simulink model "Per_MKM"  (R2019a)
settings: Solver=FixedStepDiscrete  StartTime=0.0  StopTime=50  FixedStep=1  RelTol=1e-3
undefined symbols (not defined in the file or in its folder): ADAS, ADAS_Setting, KeyPress, Setting
libraries: simulink x102
(part 1 of 2)
settings Model: DataDictionary=test2.sldd  Creator=admin  LastModifiedBy=inamdar
settings ConfigComp: CovMetricSettings=dtrzoibw  CovNameIncrementing=on  CovHtmlReporting=on  CovSaveCumulativeToWorkspaceVar=on  CovSaveSingleToWorkspaceVar=on  CovCumulativeReport=on

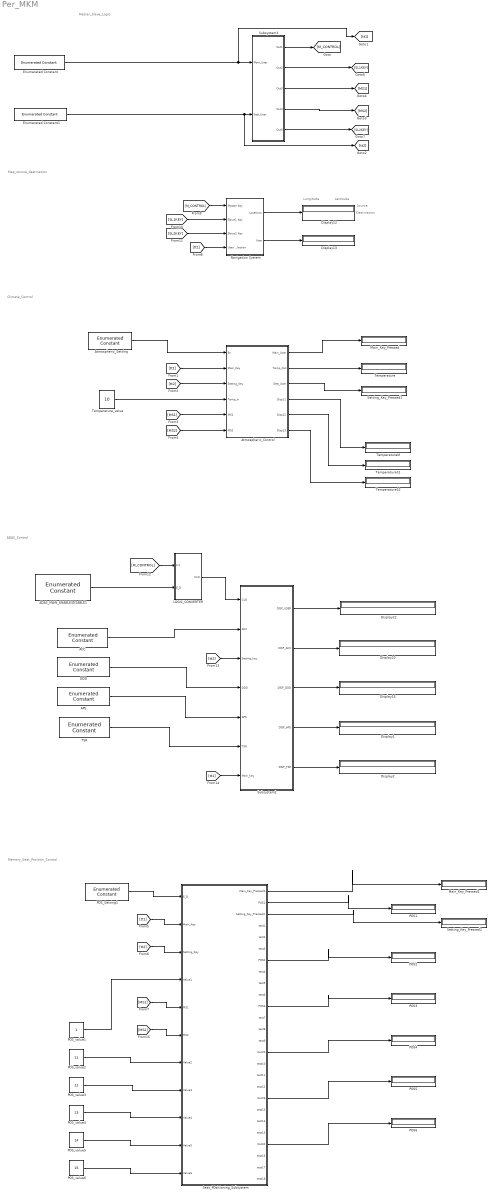
== system Per_MKM ==
  note: Memory_Seat_Position_Control
  note: Master_Slave_Logic
  note: Map_source_destination
  note: Climate_Control
  note: Longitude
  note: Lattitude
  note: Source
  note: Destination
  note: ADAS_Control
  ACC : simulink/Sources/Enumerated Constant  OutDataTypeStr=Enum: ADAS_Setting  Value=ADAS_Setting.Enable  SampleTime=inf
      settings: SourceProductName=Simulink
  ADAS_MAIN_ENABLE/DISABLE1 : simulink/Sources/Enumerated Constant  OutDataTypeStr=Enum: ADAS_Setting  Value=ADAS_Setting.Enable  SampleTime=inf
      settings: SourceProductName=Simulink
  APS : simulink/Sources/Enumerated Constant  OutDataTypeStr=Enum: ADAS_Setting  Value=ADAS_Setting.Enable  SampleTime=inf
      settings: SourceProductName=Simulink
  Atmospheric_Control : Subsystem
  Atmospheric_Setting : simulink/Sources/Enumerated Constant  OutDataTypeStr=Enum: Setting  Value=Setting.Disable  SampleTime=inf
      settings: SourceProductName=Simulink
  DDD : simulink/Sources/Enumerated Constant  OutDataTypeStr=Enum: ADAS_Setting  Value=ADAS_Setting.Enable  SampleTime=inf
      settings: SourceProductName=Simulink
  Display{1..2,12..14,20,22} (7 alike) : Display
  Enumerated Constant : simulink/Sources/Enumerated Constant  OutDataTypeStr=Enum: KeyPress  Value=KeyPress.Master  SampleTime=inf
      settings: SourceProductName=Simulink
  Enumerated Constant1 : simulink/Sources/Enumerated Constant  OutDataTypeStr=Enum: KeyPress  Value=KeyPress.Master  SampleTime=inf
      settings: SourceProductName=Simulink
  LOGIC_CONVERTER : Subsystem
  Main_Key_Pressed : Display
  Main_Key_Pressed1 : Display
  Navigation System : Subsystem
  POS{1..6} (6 alike) : Display
  POS_Setting1 : simulink/Sources/Enumerated Constant  OutDataTypeStr=Enum: Setting  Value=Setting.Disable  SampleTime=inf
      settings: SourceProductName=Simulink
  POS_value1 : Constant  OutDataTypeStr=uint8
  POS_value2 : Constant  Value=11  OutDataTypeStr=uint8
  POS_value3 : Constant  Value=12  OutDataTypeStr=uint8
  POS_value4 : Constant  Value=13  OutDataTypeStr=uint8
  POS_value5 : Constant  Value=14  OutDataTypeStr=uint8
  POS_value6 : Constant  Value=15  OutDataTypeStr=uint8
  Seat_POsitioning_Subsystem : Subsystem
  Setting_Key_Pressed1 : Display
  Setting_Key_Pressed2 : Display
  Subsystem2 : Subsystem
  Subsystem3 : Subsystem
  TSR : simulink/Sources/Enumerated Constant  OutDataTypeStr=Enum: ADAS_Setting  Value=ADAS_Setting.Enable  SampleTime=inf
      settings: SourceProductName=Simulink
  Temperature : Display
  TemperatureM : Display
  TemperatureS1 : Display
  TemperatureS2 : Display
  Temperature_value : Constant  Value=10  OutDataTypeStr=uint8
  wires:
  Enumerated Constant1/1 -> [tt2], Subsystem3/2(Sett_User)
  Navigation System/1(Locations) -> Display12/1
  Navigation System/2(User) -> Display13/1
  Enumerated Constant/1 -> [tt1], Subsystem3/1(Main_User)
  Atmospheric_Setting/1 -> Atmospheric_Control/1(En)
  [tt1] -> Atmospheric_Control/2(Main_Key)
  [tt2] -> Atmospheric_Control/3(Setting_Key)
  Temperature_value/1 -> Atmospheric_Control/4(Temp_In)
  Atmospheric_Control/1(Main_User) -> Main_Key_Pressed/1
  Atmospheric_Control/2(Temp_Out) -> Temperature/1
  Atmospheric_Control/3(Sett_User) -> Setting_Key_Pressed1/1
  [MS1] -> Atmospheric_Control/5("MS1 ")
  [MS2] -> Atmospheric_Control/6(MS2)
  [tt1] -> Navigation System/4(User Selection)
  [M_CONTROL] -> Navigation System/1("Master Key ")
  [SL1KEY] -> Navigation System/2(Slave1 Key)
  [SL2KEY] -> Navigation System/3(Slave2 Key)
  Subsystem2/5(DISP_TSR) -> Display2/1
  Subsystem2/4(DISP_APS) -> Display1/1
  Subsystem2/3(DISP_DDD) -> Display14/1
  Subsystem2/1(DISP_USER) -> Display22/1
  Subsystem2/2(DISP_ACC) -> Display20/1
  [tt1] -> Subsystem2/7(Main_key)
  TSR/1 -> Subsystem2/6(TSR)
  APS/1 -> Subsystem2/5(APS)
  DDD/1 -> Subsystem2/4(DDD)
  [tt2] -> Subsystem2/3(Setting_key)
  ACC/1 -> Subsystem2/2(ACC)
  [M_CONTROL] -> LOGIC_CONVERTER/1(In1)
  ADAS_MAIN_ENABLE/DISABLE1/1 -> LOGIC_CONVERTER/2(E_D)
  LOGIC_CONVERTER/1(CLO) -> Subsystem2/1(CLO)
  Subsystem3/1(Out1) -> [M_CONTROL]
  Subsystem3/2(Out2) -> [SL1KEY]
  Subsystem3/3(Out3) -> [MS1]
  Subsystem3/4(Out4) -> [MS2]
  Subsystem3/5(Out5) -> [SL2KEY]
  Atmospheric_Control/4(Disp11) -> TemperatureM/1
  Atmospheric_Control/5(Disp12) -> TemperatureS1/1
  Atmospheric_Control/6(Disp13) -> TemperatureS2/1
  POS_Setting1/1 -> Seat_POsitioning_Subsystem/1(E_D)
  [tt1] -> Seat_POsitioning_Subsystem/2(Main_Key)
  [tt2] -> Seat_POsitioning_Subsystem/3(Setting_Key)
  POS_value1/1 -> Seat_POsitioning_Subsystem/4(Value1)
  [MS1] -> Seat_POsitioning_Subsystem/5(MS1)
  [MS2] -> Seat_POsitioning_Subsystem/6(MS2)
  POS_value2/1 -> Seat_POsitioning_Subsystem/7(Value2)
  POS_value3/1 -> Seat_POsitioning_Subsystem/8(Value3)
  POS_value4/1 -> Seat_POsitioning_Subsystem/9(Value4)
  POS_value5/1 -> Seat_POsitioning_Subsystem/10(Value5)
  POS_value6/1 -> Seat_POsitioning_Subsystem/11(Value6)
  Seat_POsitioning_Subsystem/1(Main_Key_Pressed1) -> Main_Key_Pressed1/1
  Seat_POsitioning_Subsystem/2(POS1) -> POS1/1
  Seat_POsitioning_Subsystem/3(Setting_Key_Pressed2) -> Setting_Key_Pressed2/1
  Seat_POsitioning_Subsystem/7(POS2) -> POS2/1
  Seat_POsitioning_Subsystem/11(POS3) -> POS3/1
  Seat_POsitioning_Subsystem/15(Out20) -> POS4/1
  Seat_POsitioning_Subsystem/19(Out26) -> POS5/1
  Seat_POsitioning_Subsystem/23(Out32) -> POS6/1

== system Per_MKM/Atmospheric_Control ==
  En : Inport
  Main_Key : Inport  Port=2
  Setting_Key : Inport  Port=3
  Temp_In : Inport  Port=4
  "MS1 " : Inport  Port=5
  MS2 : Inport  Port=6
  Data Store Memory4 : DataStoreMemory  DataStoreName=TeM  ReadBeforeWriteMsg=warning  WriteAfterWriteMsg=warning  WriteAfterReadMsg=warning  ShowAdditionalParam=off  OutDataTypeStr=uint8
  Data Store Memory6 : DataStoreMemory  DataStoreName=TeS1  ReadBeforeWriteMsg=warning  WriteAfterWriteMsg=warning  WriteAfterReadMsg=warning  ShowAdditionalParam=off  OutDataTypeStr=uint8
  Data Store Memory7 : DataStoreMemory  DataStoreName=TeS2  ReadBeforeWriteMsg=warning  WriteAfterWriteMsg=warning  WriteAfterReadMsg=warning  ShowAdditionalParam=off  OutDataTypeStr=uint8
  Data Type Conversion1 : DataTypeConversion
  Data Type Conversion2 : DataTypeConversion
  Subsystem3 : Subsystem
  Subsystem4 : Subsystem
  Main_User : Outport
  Temp_Out : Outport  Port=2
  Sett_User : Outport  Port=3
  Disp11 : Outport  Port=4
  Disp12 : Outport  Port=5
  Disp13 : Outport  Port=6
  wires:
  Data Type Conversion2/1 -> Subsystem3/Enable
  Setting_Key/1 -> Subsystem3/1(In1)
  Subsystem4/1(Out1) -> Main_User/1
  Temp_In/1 -> Subsystem3/2(In2)
  Main_Key/1 -> Data Type Conversion1/1, Subsystem4/1(In1)
  Subsystem4/2(Out2) -> Temp_Out/1
  En/1 -> Data Type Conversion2/1
  MS2/1 -> Subsystem3/4(MS22)
  "MS1 "/1 -> Subsystem3/3(MS11)
  Subsystem3/1(Output) -> Sett_User/1
  Subsystem3/4(Disp3) -> Disp13/1
  Subsystem3/3(Disp2) -> Disp12/1
  Subsystem3/2(Disp1) -> Disp11/1
  Data Type Conversion1/1 -> Subsystem3/5(TT1)

== system Per_MKM/LOGIC_CONVERTER ==
  In1 : Inport
  E_D : Inport  Port=2
  AND1 : Logic  AllPortsSameDT=off  OutDataTypeStr=boolean
  Compare To Constant1 : simulink/Logic and Bit Operations/Compare To Constant  relop===  const=1  OutDataTypeStr=boolean
  Data Type Conversion2 : DataTypeConversion
  CLO : Outport
  wires:
  E_D/1 -> Data Type Conversion2/1
  Data Type Conversion2/1 -> Compare To Constant1/1
  Compare To Constant1/1 -> AND1/2
  In1/1 -> AND1/1
  AND1/1 -> CLO/1

== system Per_MKM/Navigation System ==
  "Master Key " : Inport
  Slave1 Key : Inport  Port=2
  Slave2 Key : Inport  Port=3
  User Selection : Inport  Port=4
  Subsystem2 : Subsystem
  Locations : Outport
  User : Outport  Port=2
  wires:
  "Master Key "/1 -> Subsystem2/1(In1)
  User Selection/1 -> User/1
  Slave1 Key/1 -> Subsystem2/2(In2)
  Slave2 Key/1 -> Subsystem2/3(In3)
  Subsystem2/1(Out1) -> Locations/1

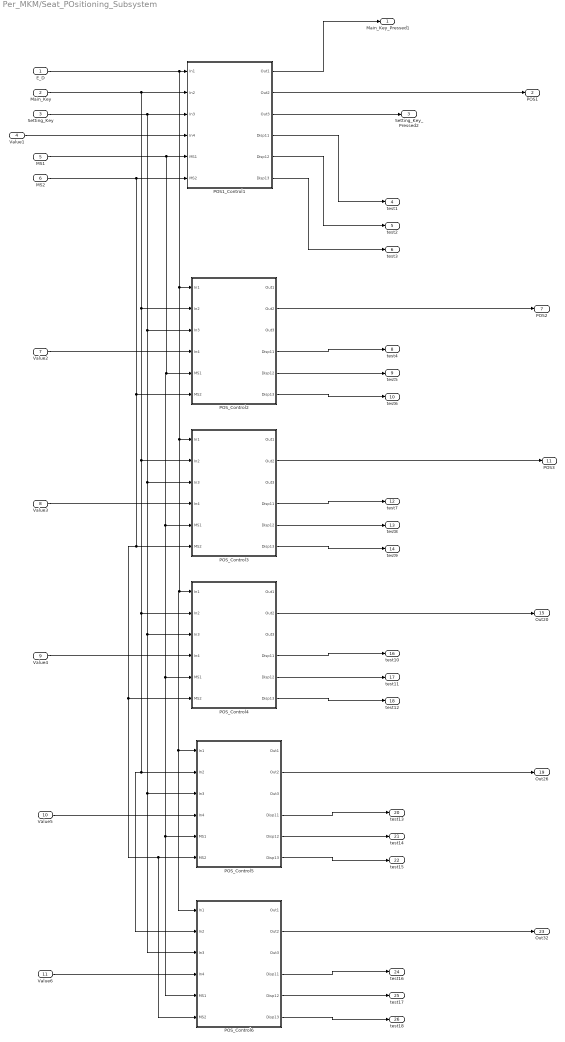
== system Per_MKM/Seat_POsitioning_Subsystem ==
  E_D : Inport
  Main_Key : Inport  Port=2
  Setting_Key : Inport  Port=3
  Value1 : Inport  Port=4
  MS1 : Inport  Port=5
  MS2 : Inport  Port=6
  Value2 : Inport  Port=7
  Value3 : Inport  Port=8
  Value4 : Inport  Port=9
  Value5 : Inport  Port=10
  Value6 : Inport  Port=11
  POS1_Control1 : Subsystem
  POS_Control2 : Subsystem
  POS_Control3 : Subsystem
  POS_Control4 : Subsystem
  POS_Control5 : Subsystem
  POS_Control6 : Subsystem
  Main_Key_Pressed1 : Outport
  POS1 : Outport  Port=2
  Setting_Key_Pressed2 : Outport  Port=3
  test1 : Outport  Port=4
  test2 : Outport  Port=5
  test3 : Outport  Port=6
  POS2 : Outport  Port=7
  test4 : Outport  Port=8
  test5 : Outport  Port=9
  test6 : Outport  Port=10
  POS3 : Outport  Port=11
  test7 : Outport  Port=12
  test8 : Outport  Port=13
  test9 : Outport  Port=14
  Out20 : Outport  Port=15
  test10 : Outport  Port=16
  test11 : Outport  Port=17
  test12 : Outport  Port=18
  Out26 : Outport  Port=19
  test13 : Outport  Port=20
  test14 : Outport  Port=21
  test15 : Outport  Port=22
  Out32 : Outport  Port=23
  test16 : Outport  Port=24
  test17 : Outport  Port=25
  test18 : Outport  Port=26
  wires:
  POS1_Control1/4(Disp11) -> test1/1
  MS1/1 -> POS_Control6/5("MS1 "), POS_Control5/5("MS1 "), POS_Control4/5("MS1 "), POS_Control3/5("MS1 "), POS_Control2/5("MS1 "), POS1_Control1/5("MS1 ")
  Setting_Key/1 -> POS_Control6/3(In3), POS_Control5/3(In3), POS_Control4/3(In3), POS_Control3/3(In3), POS_Control2/3(In3), POS1_Control1/3(In3)
  POS_Control3/4(Disp11) -> test7/1
  Main_Key/1 -> POS_Control6/2(In2), POS_Control5/2(In2), POS_Control4/2(In2), POS_Control3/2(In2), POS_Control2/2(In2), POS1_Control1/2(In2)
  E_D/1 -> POS_Control6/1(In1), POS_Control5/1(In1), POS_Control4/1(In1), POS_Control3/1(In1), POS_Control2/1(In1), POS1_Control1/1(In1)
  MS2/1 -> POS_Control6/6(MS2), POS_Control5/6(MS2), POS_Control4/6(MS2), POS_Control3/6(MS2), POS_Control2/6(MS2), POS1_Control1/6(MS2)
  Value1/1 -> POS1_Control1/4(In4)
  POS_Control6/4(Disp11) -> test16/1
  POS_Control3/6(Disp13) -> test9/1
  POS_Control3/2(Out2) -> POS3/1
  POS1_Control1/3(Out3) -> Setting_Key_Pressed2/1
  Value6/1 -> POS_Control6/4(In4)
  Value2/1 -> POS_Control2/4(In4)
  POS_Control2/5(Disp12) -> test5/1
  POS_Control2/6(Disp13) -> test6/1
  Value3/1 -> POS_Control3/4(In4)
  POS1_Control1/6(Disp13) -> test3/1
  POS1_Control1/1(Out1) -> Main_Key_Pressed1/1
  POS_Control5/5(Disp12) -> test14/1
  POS_Control5/6(Disp13) -> test15/1
  POS_Control2/2(Out2) -> POS2/1
  Value5/1 -> POS_Control5/4(In4)
  POS_Control2/4(Disp11) -> test4/1
  POS_Control3/5(Disp12) -> test8/1
  POS_Control4/4(Disp11) -> test10/1
  POS_Control4/5(Disp12) -> test11/1
  Value4/1 -> POS_Control4/4(In4)
  POS_Control6/5(Disp12) -> test17/1
  POS_Control4/6(Disp13) -> test12/1
  POS_Control5/2(Out2) -> Out26/1
  POS_Control4/2(Out2) -> Out20/1
  POS_Control6/6(Disp13) -> test18/1
  POS1_Control1/2(Out2) -> POS1/1
  POS_Control6/2(Out2) -> Out32/1
  POS1_Control1/5(Disp12) -> test2/1
  POS_Control5/4(Disp11) -> test13/1

== system Per_MKM/Subsystem2 ==
  CLO : Inport
  ACC : Inport  Port=2
  Setting_key : Inport  Port=3
  DDD : Inport  Port=4
  APS : Inport  Port=5
  TSR : Inport  Port=6
  Main_key : Inport  Port=7
  Data Store Memory : DataStoreMemory  DataStoreName=ADAS_M  ReadBeforeWriteMsg=warning  WriteAfterWriteMsg=warning  WriteAfterReadMsg=warning  ShowAdditionalParam=off
  Data Store Memory1 : DataStoreMemory  DataStoreName=ADAS_S1  ReadBeforeWriteMsg=warning  WriteAfterWriteMsg=warning  WriteAfterReadMsg=warning  ShowAdditionalParam=off
  Data Store Memory10 : DataStoreMemory  DataStoreName=ADAS_S13  ReadBeforeWriteMsg=warning  WriteAfterWriteMsg=warning  WriteAfterReadMsg=warning  ShowAdditionalParam=off
  Data Store Memory11 : DataStoreMemory  DataStoreName=ADAS_S23  ReadBeforeWriteMsg=warning  WriteAfterWriteMsg=warning  WriteAfterReadMsg=warning  ShowAdditionalParam=off
  Data Store Memory2 : DataStoreMemory  DataStoreName=ADAS_S2  ReadBeforeWriteMsg=warning  WriteAfterWriteMsg=warning  WriteAfterReadMsg=warning  ShowAdditionalParam=off
  Data Store Memory3 : DataStoreMemory  DataStoreName=ADAS_M1  ReadBeforeWriteMsg=warning  WriteAfterWriteMsg=warning  WriteAfterReadMsg=warning  ShowAdditionalParam=off
  Data Store Memory4 : DataStoreMemory  DataStoreName=ADAS_S11  ReadBeforeWriteMsg=warning  WriteAfterWriteMsg=warning  WriteAfterReadMsg=warning  ShowAdditionalParam=off
  Data Store Memory5 : DataStoreMemory  DataStoreName=ADAS_S21  ReadBeforeWriteMsg=warning  WriteAfterWriteMsg=warning  WriteAfterReadMsg=warning  ShowAdditionalParam=off
  Data Store Memory6 : DataStoreMemory  DataStoreName=ADAS_M2  ReadBeforeWriteMsg=warning  WriteAfterWriteMsg=warning  WriteAfterReadMsg=warning  ShowAdditionalParam=off
  Data Store Memory7 : DataStoreMemory  DataStoreName=ADAS_S12  ReadBeforeWriteMsg=warning  WriteAfterWriteMsg=warning  WriteAfterReadMsg=warning  ShowAdditionalParam=off
  Data Store Memory8 : DataStoreMemory  DataStoreName=ADAS_S22  ReadBeforeWriteMsg=warning  WriteAfterWriteMsg=warning  WriteAfterReadMsg=warning  ShowAdditionalParam=off
  Data Store Memory9 : DataStoreMemory  DataStoreName=ADAS_M3  ReadBeforeWriteMsg=warning  WriteAfterWriteMsg=warning  WriteAfterReadMsg=warning  ShowAdditionalParam=off
  Subsystem : Subsystem
  Subsystem1 : Subsystem
  Subsystem8 : Subsystem
  DISP_USER : Outport
  DISP_ACC : Outport  Port=2
  DISP_DDD : Outport  Port=3
  DISP_APS : Outport  Port=4
  DISP_TSR : Outport  Port=5
  wires:
  CLO/1 -> Subsystem8/Enable, [LOGIC_DISPLAY]
  TSR/1 -> Subsystem8/5(In5)
  APS/1 -> Subsystem8/4(In4)
  DDD/1 -> Subsystem8/3(In3)
  Setting_key/1 -> Subsystem8/2(In2)
  ACC/1 -> Subsystem8/1(In1)
  Main_key/1 -> Subsystem/1(In1), Subsystem1/7(In7)
  Subsystem8/1(Out1) -> Subsystem1/1(In1)
  [LOGIC_DISPLAY] -> Subsystem1/2(In2)
  Subsystem8/2(Out2) -> Subsystem1/3(In3)
  Subsystem8/3(Out3) -> Subsystem1/4(In4)
  Subsystem8/4(Out4) -> Subsystem1/5(In5)
  Subsystem8/5(Out5) -> Subsystem1/6(In6)
  Subsystem/1(Out1) -> Subsystem1/8(In8)
  Subsystem/2(Out2) -> Subsystem1/9(In9)
  Subsystem/3(Out3) -> Subsystem1/10(In10)
  Subsystem/4(Out4) -> Subsystem1/11(In11)
  Subsystem1/1(Out1) -> DISP_USER/1
  Subsystem1/2(Out2) -> DISP_ACC/1
  Subsystem1/3(Out3) -> DISP_DDD/1
  Subsystem1/4(Out4) -> DISP_APS/1
  Subsystem1/5(Out5) -> DISP_TSR/1

== system Per_MKM/Subsystem3 ==
  Main_User : Inport
  Sett_User : Inport  Port=2
  Logics : Subsystem
  Subsystem : Subsystem
  Subsystem1 : Subsystem
  Out1 : Outport
  Out2 : Outport  Port=2
  Out3 : Outport  Port=3
  Out4 : Outport  Port=4
  Out5 : Outport  Port=5
  wires:
  Subsystem1/2(Out3) -> Logics/3(In5)
  Logics/1(Out2) -> Out3/1
  Subsystem1/1(Out2) -> Logics/2(In4)
  Subsystem/2(Out3) -> Out2/1
  Subsystem/3(Out4) -> Out5/1
  Subsystem1/3(Out4) -> Logics/4(In6)
  Subsystem/1(Out2) -> Out1/1, Logics/1(In1)
  Logics/2(Out3) -> Out4/1
  Sett_User/1 -> Subsystem1/1(In1)
  Main_User/1 -> Subsystem/1(In1)

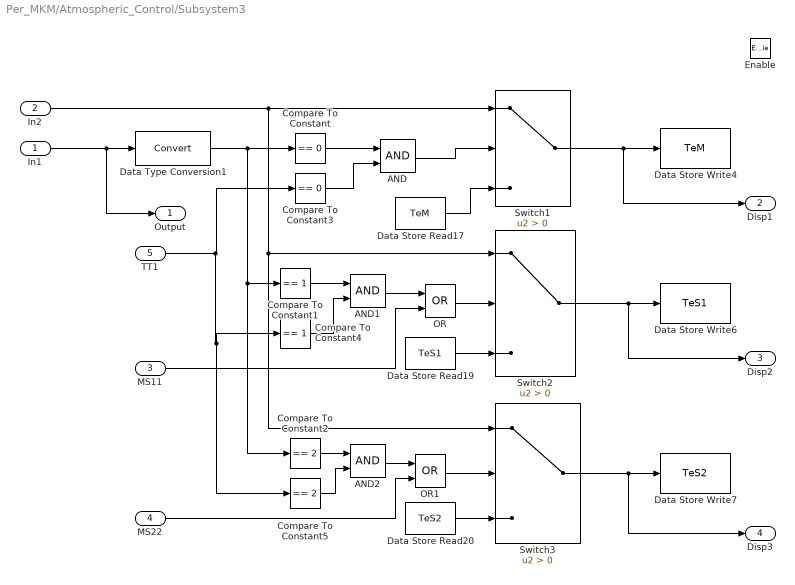
== system Per_MKM/Atmospheric_Control/Subsystem3 ==
  In1 : Inport
  In2 : Inport  Port=2
  MS11 : Inport  Port=3
  MS22 : Inport  Port=4
  TT1 : Inport  Port=5
  Enable : EnablePort
  AND : Logic  AllPortsSameDT=off  OutDataTypeStr=boolean
  AND1 : Logic  AllPortsSameDT=off  OutDataTypeStr=boolean
  AND2 : Logic  AllPortsSameDT=off  OutDataTypeStr=boolean
  Compare To Constant : simulink/Logic and Bit Operations/Compare To Constant  relop===  const=0  OutDataTypeStr=boolean
  Compare To Constant1 : simulink/Logic and Bit Operations/Compare To Constant  relop===  const=1  OutDataTypeStr=boolean
  Compare To Constant2 : simulink/Logic and Bit Operations/Compare To Constant  relop===  const=2  OutDataTypeStr=boolean
  Compare To Constant3 : simulink/Logic and Bit Operations/Compare To Constant  relop===  const=0  OutDataTypeStr=boolean
  Compare To Constant4 : simulink/Logic and Bit Operations/Compare To Constant  relop===  const=1  OutDataTypeStr=boolean
  Compare To Constant5 : simulink/Logic and Bit Operations/Compare To Constant  relop===  const=2  OutDataTypeStr=boolean
  Data Store Read17 : DataStoreRead  DataStoreName=TeM
  Data Store Read19 : DataStoreRead  DataStoreName=TeS1
  Data Store Read20 : DataStoreRead  DataStoreName=TeS2
  Data Store Write4 : DataStoreWrite  DataStoreName=TeM
  Data Store Write6 : DataStoreWrite  DataStoreName=TeS1
  Data Store Write7 : DataStoreWrite  DataStoreName=TeS2
  Data Type Conversion1 : DataTypeConversion
  OR : Logic  Operator=OR  AllPortsSameDT=off  OutDataTypeStr=boolean
  OR1 : Logic  Operator=OR  AllPortsSameDT=off  OutDataTypeStr=boolean
  Switch1 : Switch  Criteria=u2 > Threshold
  Switch2 : Switch  Criteria=u2 > Threshold
  Switch3 : Switch  Criteria=u2 > Threshold
  Output : Outport
  Disp1 : Outport  Port=2
  Disp2 : Outport  Port=3
  Disp3 : Outport  Port=4
  wires:
  Data Type Conversion1/1 -> Compare To Constant/1, Compare To Constant2/1, Compare To Constant1/1
  Switch2/1 -> Disp2/1, Data Store Write6/1
  Data Store Read20/1 -> Switch3/3
  Switch3/1 -> Disp3/1, Data Store Write7/1
  Switch1/1 -> Disp1/1, Data Store Write4/1
  Data Store Read19/1 -> Switch2/3
  Data Store Read17/1 -> Switch1/3
  In1/1 -> Output/1, Data Type Conversion1/1
  In2/1 -> Switch1/1, Switch2/1, Switch3/1
  OR/1 -> Switch2/2
  OR1/1 -> Switch3/2
  MS11/1 -> OR/2
  MS22/1 -> OR1/2
  AND/1 -> Switch1/2
  Compare To Constant/1 -> AND/1
  Compare To Constant3/1 -> AND/2
  TT1/1 -> Compare To Constant5/1, Compare To Constant4/1, Compare To Constant3/1
  Compare To Constant1/1 -> AND1/1
  Compare To Constant4/1 -> AND1/2
  AND1/1 -> OR/1
  AND2/1 -> OR1/1
  Compare To Constant2/1 -> AND2/1
  Compare To Constant5/1 -> AND2/2

== system Per_MKM/Atmospheric_Control/Subsystem4 ==
  In1 : Inport
  Data Store Read14 : DataStoreRead  DataStoreName=TeM
  Data Store Read15 : DataStoreRead  DataStoreName=TeS1
  Data Store Read16 : DataStoreRead  DataStoreName=TeS2
  Data Type Conversion : DataTypeConversion
  Multiport Switch3 : MultiPortSwitch  DataPortOrder=Zero-based contiguous  DataPortForDefault=Additional data port  zeroidx=on
  Out1 : Outport
  Out2 : Outport  Port=2
  wires:
  In1/1 -> Out1/1, Data Type Conversion/1
  Data Store Read14/1 -> Multiport Switch3/5, Multiport Switch3/2
  Multiport Switch3/1 -> Out2/1
  Data Type Conversion/1 -> Multiport Switch3/1
  Data Store Read15/1 -> Multiport Switch3/3
  Data Store Read16/1 -> Multiport Switch3/4

== system Per_MKM/Navigation System/Subsystem2 ==
  In1 : Inport
  In2 : Inport  Port=2
  In3 : Inport  Port=3
  Constant10 : Constant  Value=0
  Constant6 : Constant  Value=[18.6 73.75]
  Constant7 : Constant  Value=[18.44 73.86]
  Constant8 : Constant  Value=[ 18.43 73.77]
  Constant9 : Constant  Value=[18.53 73.87]
  Mux : Mux  Inputs=2
  Switch1 : Switch  Criteria=u2 > Threshold
  Switch2 : Switch  Criteria=u2 > Threshold
  Switch3 : Switch  Criteria=u2 > Threshold
  Out1 : Outport
  wires:
  Switch2/1 -> Switch1/3
  Constant7/1 -> Switch2/1
  Switch3/1 -> Switch2/3
  Constant9/1 -> Switch1/1
  Constant8/1 -> Switch3/1
  Constant6/1 -> Mux/1
  Switch1/1 -> Mux/2
  Constant10/1 -> Switch3/3
  In3/1 -> Switch3/2
  In2/1 -> Switch2/2
  In1/1 -> Switch1/2
  Mux/1 -> Out1/1

== system Per_MKM/Seat_POsitioning_Subsystem/POS1_Control1 ==
  In1 : Inport
  In2 : Inport  Port=2
  In3 : Inport  Port=3
  In4 : Inport  Port=4
  "MS1 " : Inport  Port=5
  MS2 : Inport  Port=6
  Data Store Memory4 : DataStoreMemory  DataStoreName=POS_M  ReadBeforeWriteMsg=warning  WriteAfterWriteMsg=warning  WriteAfterReadMsg=warning  ShowAdditionalParam=off  OutDataTypeStr=uint8
  Data Store Memory6 : DataStoreMemory  DataStoreName=POS_S1  ReadBeforeWriteMsg=warning  WriteAfterWriteMsg=warning  WriteAfterReadMsg=warning  ShowAdditionalParam=off  OutDataTypeStr=uint8
  Data Store Memory7 : DataStoreMemory  DataStoreName=POS_S2  ReadBeforeWriteMsg=warning  WriteAfterWriteMsg=warning  WriteAfterReadMsg=warning  ShowAdditionalParam=off  OutDataTypeStr=uint8
  Data Type Conversion1 : DataTypeConversion
  Data Type Conversion2 : DataTypeConversion
  Subsystem3 : Subsystem
  Subsystem4 : Subsystem
  Out1 : Outport
  Out2 : Outport  Port=2
  Out3 : Outport  Port=3
  Disp11 : Outport  Port=4
  Disp12 : Outport  Port=5
  Disp13 : Outport  Port=6
  wires:
  Data Type Conversion1/1 -> Subsystem3/5(TT1)
  Subsystem3/2(Disp1) -> Disp11/1
  Subsystem3/3(Disp2) -> Disp12/1
  Subsystem3/4(Disp3) -> Disp13/1
  Subsystem3/1(Output) -> Out3/1
  "MS1 "/1 -> Subsystem3/3(MS11)
  MS2/1 -> Subsystem3/4(MS22)
  In1/1 -> Data Type Conversion2/1
  Subsystem4/2(Out2) -> Out2/1
  In2/1 -> Subsystem4/1(In1), Data Type Conversion1/1
  In4/1 -> Subsystem3/2(In2)
  Subsystem4/1(Out1) -> Out1/1
  In3/1 -> Subsystem3/1(In1)
  Data Type Conversion2/1 -> Subsystem3/Enable

== system Per_MKM/Seat_POsitioning_Subsystem/POS_Control2 ==
  In1 : Inport
  In2 : Inport  Port=2
  In3 : Inport  Port=3
  In4 : Inport  Port=4
  "MS1 " : Inport  Port=5
  MS2 : Inport  Port=6
  Data Store Memory4 : DataStoreMemory  DataStoreName=POS_M1  ReadBeforeWriteMsg=warning  WriteAfterWriteMsg=warning  WriteAfterReadMsg=warning  ShowAdditionalParam=off  OutDataTypeStr=uint8
  Data Store Memory6 : DataStoreMemory  DataStoreName=POS_S11  ReadBeforeWriteMsg=warning  WriteAfterWriteMsg=warning  WriteAfterReadMsg=warning  ShowAdditionalParam=off  OutDataTypeStr=uint8
  Data Store Memory7 : DataStoreMemory  DataStoreName=POS_S21  ReadBeforeWriteMsg=warning  WriteAfterWriteMsg=warning  WriteAfterReadMsg=warning  ShowAdditionalParam=off  OutDataTypeStr=uint8
  Data Type Conversion1 : DataTypeConversion
  Data Type Conversion2 : DataTypeConversion
  Subsystem3 : Subsystem
  Subsystem4 : Subsystem
  Out1 : Outport
  Out2 : Outport  Port=2
  Out3 : Outport  Port=3
  Disp11 : Outport  Port=4
  Disp12 : Outport  Port=5
  Disp13 : Outport  Port=6
  wires:
  Data Type Conversion2/1 -> Subsystem3/Enable
  In3/1 -> Subsystem3/1(In1)
  Subsystem4/1(Out1) -> Out1/1
  In4/1 -> Subsystem3/2(In2)
  In2/1 -> Data Type Conversion1/1, Subsystem4/1(In1)
  Subsystem4/2(Out2) -> Out2/1
  In1/1 -> Data Type Conversion2/1
  MS2/1 -> Subsystem3/4(MS22)
  "MS1 "/1 -> Subsystem3/3(MS11)
  Subsystem3/1(Output) -> Out3/1
  Subsystem3/4(Disp3) -> Disp13/1
  Subsystem3/3(Disp2) -> Disp12/1
  Subsystem3/2(Disp1) -> Disp11/1
  Data Type Conversion1/1 -> Subsystem3/5(TT1)

== system Per_MKM/Seat_POsitioning_Subsystem/POS_Control3 ==
  In1 : Inport
  In2 : Inport  Port=2
  In3 : Inport  Port=3
  In4 : Inport  Port=4
  "MS1 " : Inport  Port=5
  MS2 : Inport  Port=6
  Data Store Memory4 : DataStoreMemory  DataStoreName=POS_M11  ReadBeforeWriteMsg=warning  WriteAfterWriteMsg=warning  WriteAfterReadMsg=warning  ShowAdditionalParam=off  OutDataTypeStr=uint8
  Data Store Memory6 : DataStoreMemory  DataStoreName=POS_S111  ReadBeforeWriteMsg=warning  WriteAfterWriteMsg=warning  WriteAfterReadMsg=warning  ShowAdditionalParam=off  OutDataTypeStr=uint8
  Data Store Memory7 : DataStoreMemory  DataStoreName=POS_S211  ReadBeforeWriteMsg=warning  WriteAfterWriteMsg=warning  WriteAfterReadMsg=warning  ShowAdditionalParam=off  OutDataTypeStr=uint8
  Data Type Conversion1 : DataTypeConversion
  Data Type Conversion2 : DataTypeConversion
  Subsystem3 : Subsystem
  Subsystem4 : Subsystem
  Out1 : Outport
  Out2 : Outport  Port=2
  Out3 : Outport  Port=3
  Disp11 : Outport  Port=4
  Disp12 : Outport  Port=5
  Disp13 : Outport  Port=6
  wires:
  Data Type Conversion1/1 -> Subsystem3/5(TT1)
  Subsystem3/2(Disp1) -> Disp11/1
  Subsystem3/3(Disp2) -> Disp12/1
  Subsystem3/4(Disp3) -> Disp13/1
  Subsystem3/1(Output) -> Out3/1
  "MS1 "/1 -> Subsystem3/3(MS11)
  MS2/1 -> Subsystem3/4(MS22)
  In1/1 -> Data Type Conversion2/1
  Subsystem4/2(Out2) -> Out2/1
  In2/1 -> Subsystem4/1(In1), Data Type Conversion1/1
  In4/1 -> Subsystem3/2(In2)
  Subsystem4/1(Out1) -> Out1/1
  In3/1 -> Subsystem3/1(In1)
  Data Type Conversion2/1 -> Subsystem3/Enable

== system Per_MKM/Seat_POsitioning_Subsystem/POS_Control4 ==
  In1 : Inport
  In2 : Inport  Port=2
  In3 : Inport  Port=3
  In4 : Inport  Port=4
  "MS1 " : Inport  Port=5
  MS2 : Inport  Port=6
  Data Store Memory4 : DataStoreMemory  DataStoreName=POS_M4  ReadBeforeWriteMsg=warning  WriteAfterWriteMsg=warning  WriteAfterReadMsg=warning  ShowAdditionalParam=off  OutDataTypeStr=uint8
  Data Store Memory6 : DataStoreMemory  DataStoreName=POS_S14  ReadBeforeWriteMsg=warning  WriteAfterWriteMsg=warning  WriteAfterReadMsg=warning  ShowAdditionalParam=off  OutDataTypeStr=uint8
  Data Store Memory7 : DataStoreMemory  DataStoreName=POS_S24  ReadBeforeWriteMsg=warning  WriteAfterWriteMsg=warning  WriteAfterReadMsg=warning  ShowAdditionalParam=off  OutDataTypeStr=uint8
  Data Type Conversion1 : DataTypeConversion
  Data Type Conversion2 : DataTypeConversion
  Subsystem3 : Subsystem
  Subsystem4 : Subsystem
  Out1 : Outport
  Out2 : Outport  Port=2
  Out3 : Outport  Port=3
  Disp11 : Outport  Port=4
  Disp12 : Outport  Port=5
  Disp13 : Outport  Port=6
  wires:
  Data Type Conversion2/1 -> Subsystem3/Enable
  In3/1 -> Subsystem3/1(In1)
  Subsystem4/1(Out1) -> Out1/1
  In4/1 -> Subsystem3/2(In2)
  In2/1 -> Data Type Conversion1/1, Subsystem4/1(In1)
  Subsystem4/2(Out2) -> Out2/1
  In1/1 -> Data Type Conversion2/1
  MS2/1 -> Subsystem3/4(MS22)
  "MS1 "/1 -> Subsystem3/3(MS11)
  Subsystem3/1(Output) -> Out3/1
  Subsystem3/4(Disp3) -> Disp13/1
  Subsystem3/3(Disp2) -> Disp12/1
  Subsystem3/2(Disp1) -> Disp11/1
  Data Type Conversion1/1 -> Subsystem3/5(TT1)

== system Per_MKM/Seat_POsitioning_Subsystem/POS_Control5 ==
  In1 : Inport
  In2 : Inport  Port=2
  In3 : Inport  Port=3
  In4 : Inport  Port=4
  "MS1 " : Inport  Port=5
  MS2 : Inport  Port=6
  Data Store Memory4 : DataStoreMemory  DataStoreName=POS_M5  ReadBeforeWriteMsg=warning  WriteAfterWriteMsg=warning  WriteAfterReadMsg=warning  ShowAdditionalParam=off  OutDataTypeStr=uint8
  Data Store Memory6 : DataStoreMemory  DataStoreName=POS_S15  ReadBeforeWriteMsg=warning  WriteAfterWriteMsg=warning  WriteAfterReadMsg=warning  ShowAdditionalParam=off  OutDataTypeStr=uint8
  Data Store Memory7 : DataStoreMemory  DataStoreName=POS_S25  ReadBeforeWriteMsg=warning  WriteAfterWriteMsg=warning  WriteAfterReadMsg=warning  ShowAdditionalParam=off  OutDataTypeStr=uint8
  Data Type Conversion1 : DataTypeConversion
  Data Type Conversion2 : DataTypeConversion
  Subsystem3 : Subsystem
  Subsystem4 : Subsystem
  Out1 : Outport
  Out2 : Outport  Port=2
  Out3 : Outport  Port=3
  Disp11 : Outport  Port=4
  Disp12 : Outport  Port=5
  Disp13 : Outport  Port=6
  wires:
  Data Type Conversion1/1 -> Subsystem3/5(TT1)
  Subsystem3/2(Disp1) -> Disp11/1
  Subsystem3/3(Disp2) -> Disp12/1
  Subsystem3/4(Disp3) -> Disp13/1
  Subsystem3/1(Output) -> Out3/1
  "MS1 "/1 -> Subsystem3/3(MS11)
  MS2/1 -> Subsystem3/4(MS22)
  In1/1 -> Data Type Conversion2/1
  Subsystem4/2(Out2) -> Out2/1
  In2/1 -> Subsystem4/1(In1), Data Type Conversion1/1
  In4/1 -> Subsystem3/2(In2)
  Subsystem4/1(Out1) -> Out1/1
  In3/1 -> Subsystem3/1(In1)
  Data Type Conversion2/1 -> Subsystem3/Enable

== system Per_MKM/Seat_POsitioning_Subsystem/POS_Control6 ==
  In1 : Inport
  In2 : Inport  Port=2
  In3 : Inport  Port=3
  In4 : Inport  Port=4
  "MS1 " : Inport  Port=5
  MS2 : Inport  Port=6
  Data Store Memory4 : DataStoreMemory  DataStoreName=POS_M6  ReadBeforeWriteMsg=warning  WriteAfterWriteMsg=warning  WriteAfterReadMsg=warning  ShowAdditionalParam=off  OutDataTypeStr=uint8
  Data Store Memory6 : DataStoreMemory  DataStoreName=POS_S16  ReadBeforeWriteMsg=warning  WriteAfterWriteMsg=warning  WriteAfterReadMsg=warning  ShowAdditionalParam=off  OutDataTypeStr=uint8
  Data Store Memory7 : DataStoreMemory  DataStoreName=POS_S26  ReadBeforeWriteMsg=warning  WriteAfterWriteMsg=warning  WriteAfterReadMsg=warning  ShowAdditionalParam=off  OutDataTypeStr=uint8
  Data Type Conversion1 : DataTypeConversion
  Data Type Conversion2 : DataTypeConversion
  Subsystem3 : Subsystem
  Subsystem4 : Subsystem
  Out1 : Outport
  Out2 : Outport  Port=2
  Out3 : Outport  Port=3
  Disp11 : Outport  Port=4
  Disp12 : Outport  Port=5
  Disp13 : Outport  Port=6
  wires:
  Data Type Conversion2/1 -> Subsystem3/Enable
  In3/1 -> Subsystem3/1(In1)
  Subsystem4/1(Out1) -> Out1/1
  In4/1 -> Subsystem3/2(In2)
  In2/1 -> Data Type Conversion1/1, Subsystem4/1(In1)
  Subsystem4/2(Out2) -> Out2/1
  In1/1 -> Data Type Conversion2/1
  MS2/1 -> Subsystem3/4(MS22)
  "MS1 "/1 -> Subsystem3/3(MS11)
  Subsystem3/1(Output) -> Out3/1
  Subsystem3/4(Disp3) -> Disp13/1
  Subsystem3/3(Disp2) -> Disp12/1
  Subsystem3/2(Disp1) -> Disp11/1
  Data Type Conversion1/1 -> Subsystem3/5(TT1)

== system Per_MKM/Subsystem2/Subsystem ==
  In1 : Inport
  Subsystem_ACC : Subsystem
  Subsystem_APSD : Subsystem
  Subsystem_DDDE : Subsystem
  Subsystem_TSRC : Subsystem
  Out1 : Outport
  Out2 : Outport  Port=2
  Out3 : Outport  Port=3
  Out4 : Outport  Port=4
  wires:
  Subsystem_ACC/1(Out1) -> Out1/1
  In1/1 -> Subsystem_TSRC/1(In1), Subsystem_APSD/1(In1), Subsystem_DDDE/1(In1), Subsystem_ACC/1(In1)
  Subsystem_DDDE/1(Out1) -> Out2/1
  Subsystem_APSD/1(Out1) -> Out3/1
  Subsystem_TSRC/1(Out1) -> Out4/1

== system Per_MKM/Subsystem2/Subsystem1 ==
  In1 : Inport
  In2 : Inport  Port=2
  In3 : Inport  Port=3
  In4 : Inport  Port=4
  In5 : Inport  Port=5
  In6 : Inport  Port=6
  In7 : Inport  Port=7
  In8 : Inport  Port=8
  In9 : Inport  Port=9
  In10 : Inport  Port=10
  In11 : Inport  Port=11
  Switch{,1..4} (5 alike) : Switch  Criteria=u2 > Threshold
  Out1 : Outport
  Out2 : Outport  Port=2
  Out3 : Outport  Port=3
  Out4 : Outport  Port=4
  Out5 : Outport  Port=5
  wires:
  In2/1 -> Switch/2, Switch1/2, Switch2/2, Switch4/2, Switch3/2
  Switch1/1 -> Out2/1
  Switch2/1 -> Out3/1
  In10/1 -> Switch3/3
  In4/1 -> Switch2/1
  In1/1 -> Switch1/1
  Switch/1 -> Out1/1
  In6/1 -> Switch4/1
  Switch4/1 -> Out5/1
  In8/1 -> Switch1/3
  In3/1 -> Switch/1
  Switch3/1 -> Out4/1
  In7/1 -> Switch/3
  In5/1 -> Switch3/1
  In9/1 -> Switch2/3
  In11/1 -> Switch4/3

== system Per_MKM/Subsystem2/Subsystem8 ==
  In1 : Inport
  In2 : Inport  Port=2
  In3 : Inport  Port=3
  In4 : Inport  Port=4
  In5 : Inport  Port=5
  Enable : EnablePort
  Subsystem3 : Subsystem
  Subsystem4 : Subsystem
  Subsystem5 : Subsystem
  Subsystem7 : Subsystem
  Out1 : Outport
  Out2 : Outport  Port=2
  Out3 : Outport  Port=3
  Out4 : Outport  Port=4
  Out5 : Outport  Port=5
  wires:
  Subsystem7/1(Out1) -> Out3/1
  Subsystem3/1(Out1) -> Out1/1
  Subsystem3/2(User_Disp) -> Out2/1
  In5/1 -> Subsystem5/1(In1)
  Subsystem4/1(Out1) -> Out4/1
  In4/1 -> Subsystem4/1(In1)
  Subsystem5/1(Out1) -> Out5/1
  In2/1 -> Subsystem3/2(key_pressed), Subsystem7/2(key_pressed), Subsystem4/2(key_pressed), Subsystem5/2(key_pressed)
  In3/1 -> Subsystem7/1(In1)
  In1/1 -> Subsystem3/1(In1)

== system Per_MKM/Subsystem3/Logics ==
  In1 : Inport
  In4 : Inport  Port=2
  In5 : Inport  Port=3
  In6 : Inport  Port=4
  AND3 : Logic  AllPortsSameDT=off  OutDataTypeStr=boolean
  AND4 : Logic  AllPortsSameDT=off  OutDataTypeStr=boolean
  Out2 : Outport
  Out3 : Outport  Port=2
  wires:
  AND4/1 -> Out3/1
  In5/1 -> AND3/2
  In6/1 -> AND4/2
  In1/1 -> AND3/1, AND4/1
  AND3/1 -> Out2/1

== system Per_MKM/Subsystem3/Subsystem ==
  In1 : Inport
  Compare To Constant : simulink/Logic and Bit Operations/Compare To Constant  relop===  const=0  OutDataTypeStr=boolean
  Compare To Constant2 : simulink/Logic and Bit Operations/Compare To Constant  relop===  const=1  OutDataTypeStr=boolean
  Compare To Constant3 : simulink/Logic and Bit Operations/Compare To Constant  relop===  const=2  OutDataTypeStr=boolean
  Data Type Conversion : DataTypeConversion
  Out2 : Outport
  Out3 : Outport  Port=2
  Out4 : Outport  Port=3
  wires:
  In1/1 -> Data Type Conversion/1
  Data Type Conversion/1 -> Compare To Constant3/1, Compare To Constant2/1, Compare To Constant/1
  Compare To Constant/1 -> Out2/1
  Compare To Constant2/1 -> Out3/1
  Compare To Constant3/1 -> Out4/1

== system Per_MKM/Subsystem3/Subsystem1 ==
  In1 : Inport
  Compare To Constant1 : simulink/Logic and Bit Operations/Compare To Constant  relop===  const=0  OutDataTypeStr=boolean
  Compare To Constant4 : simulink/Logic and Bit Operations/Compare To Constant  relop===  const=1  OutDataTypeStr=boolean
  Compare To Constant5 : simulink/Logic and Bit Operations/Compare To Constant  relop===  const=2  OutDataTypeStr=boolean
  Data Type Conversion1 : DataTypeConversion
  Out2 : Outport
  Out3 : Outport  Port=2
  Out4 : Outport  Port=3
  wires:
  Compare To Constant5/1 -> Out4/1
  Data Type Conversion1/1 -> Compare To Constant5/1, Compare To Constant4/1, Compare To Constant1/1
  Compare To Constant1/1 -> Out2/1
  In1/1 -> Data Type Conversion1/1
  Compare To Constant4/1 -> Out3/1

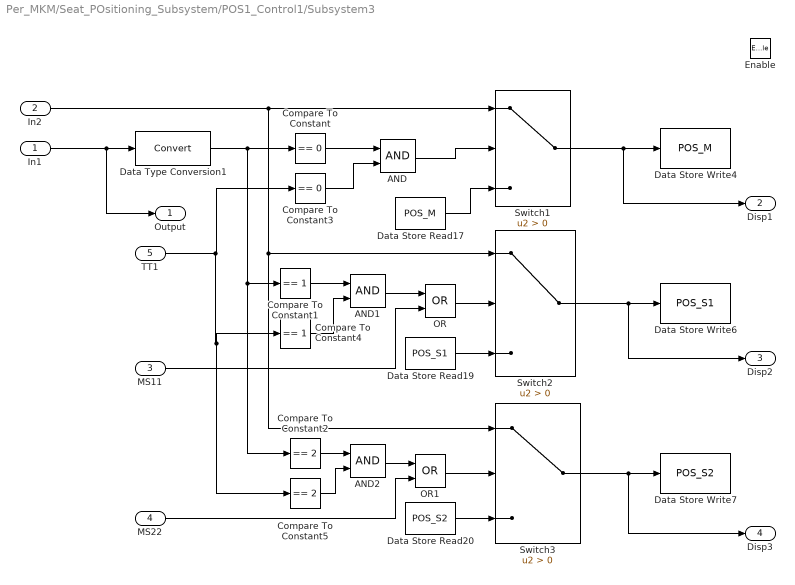
== system Per_MKM/Seat_POsitioning_Subsystem/POS1_Control1/Subsystem3 ==
  In1 : Inport
  In2 : Inport  Port=2
  MS11 : Inport  Port=3
  MS22 : Inport  Port=4
  TT1 : Inport  Port=5
  Enable : EnablePort
  AND : Logic  AllPortsSameDT=off  OutDataTypeStr=boolean
  AND1 : Logic  AllPortsSameDT=off  OutDataTypeStr=boolean
  AND2 : Logic  AllPortsSameDT=off  OutDataTypeStr=boolean
  Compare To Constant : simulink/Logic and Bit Operations/Compare To Constant  relop===  const=0  OutDataTypeStr=boolean
  Compare To Constant1 : simulink/Logic and Bit Operations/Compare To Constant  relop===  const=1  OutDataTypeStr=boolean
  Compare To Constant2 : simulink/Logic and Bit Operations/Compare To Constant  relop===  const=2  OutDataTypeStr=boolean
  Compare To Constant3 : simulink/Logic and Bit Operations/Compare To Constant  relop===  const=0  OutDataTypeStr=boolean
  Compare To Constant4 : simulink/Logic and Bit Operations/Compare To Constant  relop===  const=1  OutDataTypeStr=boolean
  Compare To Constant5 : simulink/Logic and Bit Operations/Compare To Constant  relop===  const=2  OutDataTypeStr=boolean
  Data Store Read17 : DataStoreRead  DataStoreName=POS_M
  Data Store Read19 : DataStoreRead  DataStoreName=POS_S1
  Data Store Read20 : DataStoreRead  DataStoreName=POS_S2
  Data Store Write4 : DataStoreWrite  DataStoreName=POS_M
  Data Store Write6 : DataStoreWrite  DataStoreName=POS_S1
  Data Store Write7 : DataStoreWrite  DataStoreName=POS_S2
  Data Type Conversion1 : DataTypeConversion
  OR : Logic  Operator=OR  AllPortsSameDT=off  OutDataTypeStr=boolean
  OR1 : Logic  Operator=OR  AllPortsSameDT=off  OutDataTypeStr=boolean
  Switch1 : Switch  Criteria=u2 > Threshold
  Switch2 : Switch  Criteria=u2 > Threshold
  Switch3 : Switch  Criteria=u2 > Threshold
  Output : Outport
  Disp1 : Outport  Port=2
  Disp2 : Outport  Port=3
  Disp3 : Outport  Port=4
  wires:
  Compare To Constant5/1 -> AND2/2
  Compare To Constant2/1 -> AND2/1
  AND2/1 -> OR1/1
  AND1/1 -> OR/1
  Compare To Constant4/1 -> AND1/2
  Compare To Constant1/1 -> AND1/1
  TT1/1 -> Compare To Constant3/1, Compare To Constant4/1, Compare To Constant5/1
  Compare To Constant3/1 -> AND/2
  Compare To Constant/1 -> AND/1
  AND/1 -> Switch1/2
  MS22/1 -> OR1/2
  MS11/1 -> OR/2
  OR1/1 -> Switch3/2
  OR/1 -> Switch2/2
  In2/1 -> Switch3/1, Switch2/1, Switch1/1
  In1/1 -> Data Type Conversion1/1, Output/1
  Data Store Read17/1 -> Switch1/3
  Data Store Read19/1 -> Switch2/3
  Switch1/1 -> Data Store Write4/1, Disp1/1
  Switch3/1 -> Data Store Write7/1, Disp3/1
  Data Store Read20/1 -> Switch3/3
  Switch2/1 -> Data Store Write6/1, Disp2/1
  Data Type Conversion1/1 -> Compare To Constant1/1, Compare To Constant2/1, Compare To Constant/1

== system Per_MKM/Seat_POsitioning_Subsystem/POS1_Control1/Subsystem4 ==
  In1 : Inport
  Data Store Read14 : DataStoreRead  DataStoreName=POS_M
  Data Store Read15 : DataStoreRead  DataStoreName=POS_S1
  Data Store Read16 : DataStoreRead  DataStoreName=POS_S2
  Data Type Conversion : DataTypeConversion
  Multiport Switch3 : MultiPortSwitch  DataPortOrder=Zero-based contiguous  DataPortForDefault=Additional data port  zeroidx=on
  Out1 : Outport
  Out2 : Outport  Port=2
  wires:
  Data Store Read16/1 -> Multiport Switch3/4
  Data Store Read15/1 -> Multiport Switch3/3
  Data Type Conversion/1 -> Multiport Switch3/1
  Multiport Switch3/1 -> Out2/1
  Data Store Read14/1 -> Multiport Switch3/2, Multiport Switch3/5
  In1/1 -> Data Type Conversion/1, Out1/1

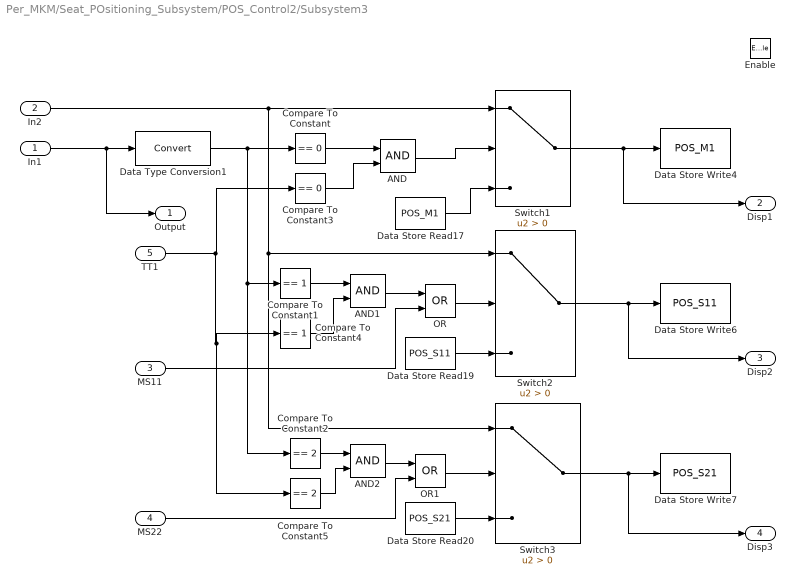
== system Per_MKM/Seat_POsitioning_Subsystem/POS_Control2/Subsystem3 ==
  In1 : Inport
  In2 : Inport  Port=2
  MS11 : Inport  Port=3
  MS22 : Inport  Port=4
  TT1 : Inport  Port=5
  Enable : EnablePort
  AND : Logic  AllPortsSameDT=off  OutDataTypeStr=boolean
  AND1 : Logic  AllPortsSameDT=off  OutDataTypeStr=boolean
  AND2 : Logic  AllPortsSameDT=off  OutDataTypeStr=boolean
  Compare To Constant : simulink/Logic and Bit Operations/Compare To Constant  relop===  const=0  OutDataTypeStr=boolean
  Compare To Constant1 : simulink/Logic and Bit Operations/Compare To Constant  relop===  const=1  OutDataTypeStr=boolean
  Compare To Constant2 : simulink/Logic and Bit Operations/Compare To Constant  relop===  const=2  OutDataTypeStr=boolean
  Compare To Constant3 : simulink/Logic and Bit Operations/Compare To Constant  relop===  const=0  OutDataTypeStr=boolean
  Compare To Constant4 : simulink/Logic and Bit Operations/Compare To Constant  relop===  const=1  OutDataTypeStr=boolean
  Compare To Constant5 : simulink/Logic and Bit Operations/Compare To Constant  relop===  const=2  OutDataTypeStr=boolean
  Data Store Read17 : DataStoreRead  DataStoreName=POS_M1
  Data Store Read19 : DataStoreRead  DataStoreName=POS_S11
  Data Store Read20 : DataStoreRead  DataStoreName=POS_S21
  Data Store Write4 : DataStoreWrite  DataStoreName=POS_M1
  Data Store Write6 : DataStoreWrite  DataStoreName=POS_S11
  Data Store Write7 : DataStoreWrite  DataStoreName=POS_S21
  Data Type Conversion1 : DataTypeConversion
  OR : Logic  Operator=OR  AllPortsSameDT=off  OutDataTypeStr=boolean
  OR1 : Logic  Operator=OR  AllPortsSameDT=off  OutDataTypeStr=boolean
  Switch1 : Switch  Criteria=u2 > Threshold
  Switch2 : Switch  Criteria=u2 > Threshold
  Switch3 : Switch  Criteria=u2 > Threshold
  Output : Outport
  Disp1 : Outport  Port=2
  Disp2 : Outport  Port=3
  Disp3 : Outport  Port=4
  wires:
  Data Type Conversion1/1 -> Compare To Constant/1, Compare To Constant2/1, Compare To Constant1/1
  Switch2/1 -> Disp2/1, Data Store Write6/1
  Data Store Read20/1 -> Switch3/3
  Switch3/1 -> Disp3/1, Data Store Write7/1
  Switch1/1 -> Disp1/1, Data Store Write4/1
  Data Store Read19/1 -> Switch2/3
  Data Store Read17/1 -> Switch1/3
  In1/1 -> Output/1, Data Type Conversion1/1
  In2/1 -> Switch1/1, Switch2/1, Switch3/1
  OR/1 -> Switch2/2
  OR1/1 -> Switch3/2
  MS11/1 -> OR/2
  MS22/1 -> OR1/2
  AND/1 -> Switch1/2
  Compare To Constant/1 -> AND/1
  Compare To Constant3/1 -> AND/2
  TT1/1 -> Compare To Constant5/1, Compare To Constant4/1, Compare To Constant3/1
  Compare To Constant1/1 -> AND1/1
  Compare To Constant4/1 -> AND1/2
  AND1/1 -> OR/1
  AND2/1 -> OR1/1
  Compare To Constant2/1 -> AND2/1
  Compare To Constant5/1 -> AND2/2

== system Per_MKM/Seat_POsitioning_Subsystem/POS_Control2/Subsystem4 ==
  In1 : Inport
  Data Store Read14 : DataStoreRead  DataStoreName=POS_M1
  Data Store Read15 : DataStoreRead  DataStoreName=POS_S11
  Data Store Read16 : DataStoreRead  DataStoreName=POS_S21
  Data Type Conversion : DataTypeConversion
  Multiport Switch3 : MultiPortSwitch  DataPortOrder=Zero-based contiguous  DataPortForDefault=Additional data port  zeroidx=on
  Out1 : Outport
  Out2 : Outport  Port=2
  wires:
  In1/1 -> Out1/1, Data Type Conversion/1
  Data Store Read14/1 -> Multiport Switch3/5, Multiport Switch3/2
  Multiport Switch3/1 -> Out2/1
  Data Type Conversion/1 -> Multiport Switch3/1
  Data Store Read15/1 -> Multiport Switch3/3
  Data Store Read16/1 -> Multiport Switch3/4

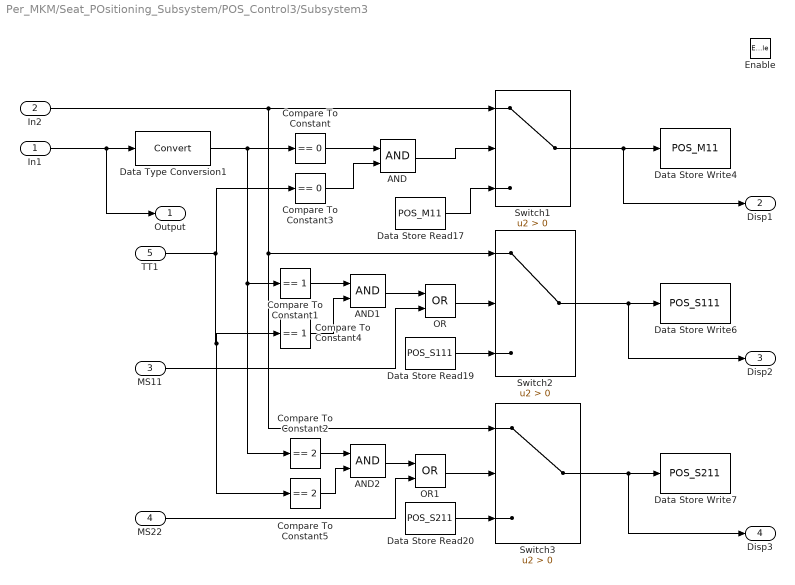
== system Per_MKM/Seat_POsitioning_Subsystem/POS_Control3/Subsystem3 ==
  In1 : Inport
  In2 : Inport  Port=2
  MS11 : Inport  Port=3
  MS22 : Inport  Port=4
  TT1 : Inport  Port=5
  Enable : EnablePort
  AND : Logic  AllPortsSameDT=off  OutDataTypeStr=boolean
  AND1 : Logic  AllPortsSameDT=off  OutDataTypeStr=boolean
  AND2 : Logic  AllPortsSameDT=off  OutDataTypeStr=boolean
  Compare To Constant : simulink/Logic and Bit Operations/Compare To Constant  relop===  const=0  OutDataTypeStr=boolean
  Compare To Constant1 : simulink/Logic and Bit Operations/Compare To Constant  relop===  const=1  OutDataTypeStr=boolean
  Compare To Constant2 : simulink/Logic and Bit Operations/Compare To Constant  relop===  const=2  OutDataTypeStr=boolean
  Compare To Constant3 : simulink/Logic and Bit Operations/Compare To Constant  relop===  const=0  OutDataTypeStr=boolean
  Compare To Constant4 : simulink/Logic and Bit Operations/Compare To Constant  relop===  const=1  OutDataTypeStr=boolean
  Compare To Constant5 : simulink/Logic and Bit Operations/Compare To Constant  relop===  const=2  OutDataTypeStr=boolean
  Data Store Read17 : DataStoreRead  DataStoreName=POS_M11
  Data Store Read19 : DataStoreRead  DataStoreName=POS_S111
  Data Store Read20 : DataStoreRead  DataStoreName=POS_S211
  Data Store Write4 : DataStoreWrite  DataStoreName=POS_M11
  Data Store Write6 : DataStoreWrite  DataStoreName=POS_S111
  Data Store Write7 : DataStoreWrite  DataStoreName=POS_S211
  Data Type Conversion1 : DataTypeConversion
  OR : Logic  Operator=OR  AllPortsSameDT=off  OutDataTypeStr=boolean
  OR1 : Logic  Operator=OR  AllPortsSameDT=off  OutDataTypeStr=boolean
  Switch1 : Switch  Criteria=u2 > Threshold
  Switch2 : Switch  Criteria=u2 > Threshold
  Switch3 : Switch  Criteria=u2 > Threshold
  Output : Outport
  Disp1 : Outport  Port=2
  Disp2 : Outport  Port=3
  Disp3 : Outport  Port=4
  wires:
  Compare To Constant5/1 -> AND2/2
  Compare To Constant2/1 -> AND2/1
  AND2/1 -> OR1/1
  AND1/1 -> OR/1
  Compare To Constant4/1 -> AND1/2
  Compare To Constant1/1 -> AND1/1
  TT1/1 -> Compare To Constant3/1, Compare To Constant4/1, Compare To Constant5/1
  Compare To Constant3/1 -> AND/2
  Compare To Constant/1 -> AND/1
  AND/1 -> Switch1/2
  MS22/1 -> OR1/2
  MS11/1 -> OR/2
  OR1/1 -> Switch3/2
  OR/1 -> Switch2/2
  In2/1 -> Switch3/1, Switch2/1, Switch1/1
  In1/1 -> Data Type Conversion1/1, Output/1
  Data Store Read17/1 -> Switch1/3
  Data Store Read19/1 -> Switch2/3
  Switch1/1 -> Data Store Write4/1, Disp1/1
  Switch3/1 -> Data Store Write7/1, Disp3/1
  Data Store Read20/1 -> Switch3/3
  Switch2/1 -> Data Store Write6/1, Disp2/1
  Data Type Conversion1/1 -> Compare To Constant1/1, Compare To Constant2/1, Compare To Constant/1

== system Per_MKM/Seat_POsitioning_Subsystem/POS_Control3/Subsystem4 ==
  In1 : Inport
  Data Store Read14 : DataStoreRead  DataStoreName=POS_M11
  Data Store Read15 : DataStoreRead  DataStoreName=POS_S111
  Data Store Read16 : DataStoreRead  DataStoreName=POS_S211
  Data Type Conversion : DataTypeConversion
  Multiport Switch3 : MultiPortSwitch  DataPortOrder=Zero-based contiguous  DataPortForDefault=Additional data port  zeroidx=on
  Out1 : Outport
  Out2 : Outport  Port=2
  wires:
  Data Store Read16/1 -> Multiport Switch3/4
  Data Store Read15/1 -> Multiport Switch3/3
  Data Type Conversion/1 -> Multiport Switch3/1
  Multiport Switch3/1 -> Out2/1
  Data Store Read14/1 -> Multiport Switch3/2, Multiport Switch3/5
  In1/1 -> Data Type Conversion/1, Out1/1

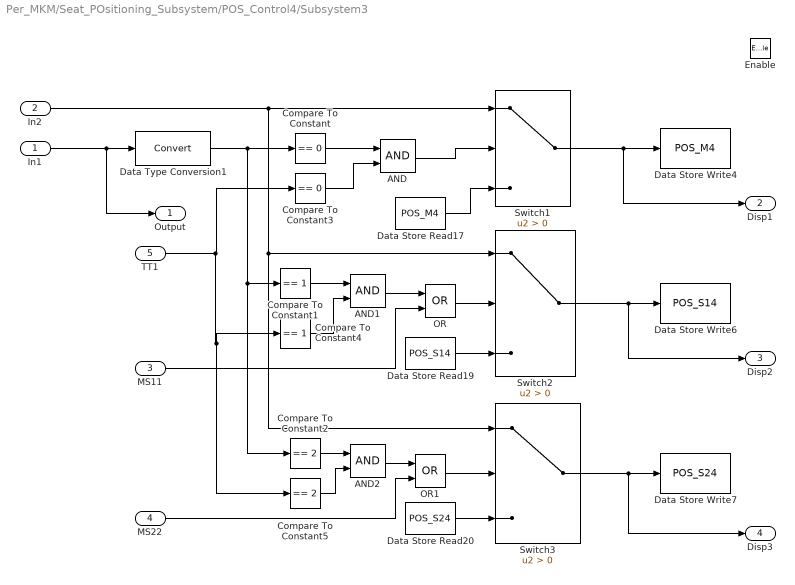
== system Per_MKM/Seat_POsitioning_Subsystem/POS_Control4/Subsystem3 ==
  In1 : Inport
  In2 : Inport  Port=2
  MS11 : Inport  Port=3
  MS22 : Inport  Port=4
  TT1 : Inport  Port=5
  Enable : EnablePort
  AND : Logic  AllPortsSameDT=off  OutDataTypeStr=boolean
  AND1 : Logic  AllPortsSameDT=off  OutDataTypeStr=boolean
  AND2 : Logic  AllPortsSameDT=off  OutDataTypeStr=boolean
  Compare To Constant : simulink/Logic and Bit Operations/Compare To Constant  relop===  const=0  OutDataTypeStr=boolean
  Compare To Constant1 : simulink/Logic and Bit Operations/Compare To Constant  relop===  const=1  OutDataTypeStr=boolean
  Compare To Constant2 : simulink/Logic and Bit Operations/Compare To Constant  relop===  const=2  OutDataTypeStr=boolean
  Compare To Constant3 : simulink/Logic and Bit Operations/Compare To Constant  relop===  const=0  OutDataTypeStr=boolean
  Compare To Constant4 : simulink/Logic and Bit Operations/Compare To Constant  relop===  const=1  OutDataTypeStr=boolean
  Compare To Constant5 : simulink/Logic and Bit Operations/Compare To Constant  relop===  const=2  OutDataTypeStr=boolean
  Data Store Read17 : DataStoreRead  DataStoreName=POS_M4
  Data Store Read19 : DataStoreRead  DataStoreName=POS_S14
  Data Store Read20 : DataStoreRead  DataStoreName=POS_S24
  Data Store Write4 : DataStoreWrite  DataStoreName=POS_M4
  Data Store Write6 : DataStoreWrite  DataStoreName=POS_S14
  Data Store Write7 : DataStoreWrite  DataStoreName=POS_S24
  Data Type Conversion1 : DataTypeConversion
  OR : Logic  Operator=OR  AllPortsSameDT=off  OutDataTypeStr=boolean
  OR1 : Logic  Operator=OR  AllPortsSameDT=off  OutDataTypeStr=boolean
  Switch1 : Switch  Criteria=u2 > Threshold
  Switch2 : Switch  Criteria=u2 > Threshold
  Switch3 : Switch  Criteria=u2 > Threshold
  Output : Outport
  Disp1 : Outport  Port=2
  Disp2 : Outport  Port=3
  Disp3 : Outport  Port=4
  wires:
  Data Type Conversion1/1 -> Compare To Constant/1, Compare To Constant2/1, Compare To Constant1/1
  Switch2/1 -> Disp2/1, Data Store Write6/1
  Data Store Read20/1 -> Switch3/3
  Switch3/1 -> Disp3/1, Data Store Write7/1
  Switch1/1 -> Disp1/1, Data Store Write4/1
  Data Store Read19/1 -> Switch2/3
  Data Store Read17/1 -> Switch1/3
  In1/1 -> Output/1, Data Type Conversion1/1
  In2/1 -> Switch1/1, Switch2/1, Switch3/1
  OR/1 -> Switch2/2
  OR1/1 -> Switch3/2
  MS11/1 -> OR/2
  MS22/1 -> OR1/2
  AND/1 -> Switch1/2
  Compare To Constant/1 -> AND/1
  Compare To Constant3/1 -> AND/2
  TT1/1 -> Compare To Constant5/1, Compare To Constant4/1, Compare To Constant3/1
  Compare To Constant1/1 -> AND1/1
  Compare To Constant4/1 -> AND1/2
  AND1/1 -> OR/1
  AND2/1 -> OR1/1
  Compare To Constant2/1 -> AND2/1
  Compare To Constant5/1 -> AND2/2

== system Per_MKM/Seat_POsitioning_Subsystem/POS_Control4/Subsystem4 ==
  In1 : Inport
  Data Store Read14 : DataStoreRead  DataStoreName=POS_M4
  Data Store Read15 : DataStoreRead  DataStoreName=POS_S14
  Data Store Read16 : DataStoreRead  DataStoreName=POS_S24
  Data Type Conversion : DataTypeConversion
  Multiport Switch3 : MultiPortSwitch  DataPortOrder=Zero-based contiguous  DataPortForDefault=Additional data port  zeroidx=on
  Out1 : Outport
  Out2 : Outport  Port=2
  wires:
  In1/1 -> Out1/1, Data Type Conversion/1
  Data Store Read14/1 -> Multiport Switch3/5, Multiport Switch3/2
  Multiport Switch3/1 -> Out2/1
  Data Type Conversion/1 -> Multiport Switch3/1
  Data Store Read15/1 -> Multiport Switch3/3
  Data Store Read16/1 -> Multiport Switch3/4

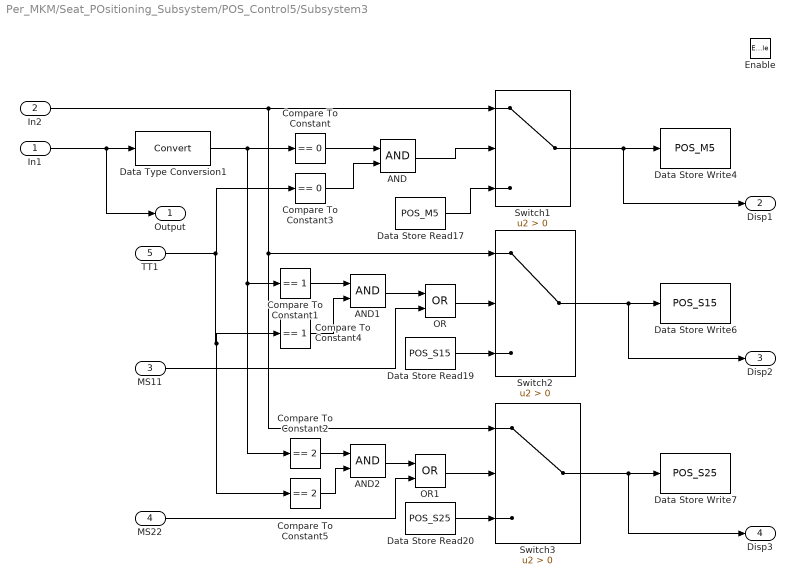
== system Per_MKM/Seat_POsitioning_Subsystem/POS_Control5/Subsystem3 ==
  In1 : Inport
  In2 : Inport  Port=2
  MS11 : Inport  Port=3
  MS22 : Inport  Port=4
  TT1 : Inport  Port=5
  Enable : EnablePort
  AND : Logic  AllPortsSameDT=off  OutDataTypeStr=boolean
  AND1 : Logic  AllPortsSameDT=off  OutDataTypeStr=boolean
  AND2 : Logic  AllPortsSameDT=off  OutDataTypeStr=boolean
  Compare To Constant : simulink/Logic and Bit Operations/Compare To Constant  relop===  const=0  OutDataTypeStr=boolean
  Compare To Constant1 : simulink/Logic and Bit Operations/Compare To Constant  relop===  const=1  OutDataTypeStr=boolean
  Compare To Constant2 : simulink/Logic and Bit Operations/Compare To Constant  relop===  const=2  OutDataTypeStr=boolean
  Compare To Constant3 : simulink/Logic and Bit Operations/Compare To Constant  relop===  const=0  OutDataTypeStr=boolean
  Compare To Constant4 : simulink/Logic and Bit Operations/Compare To Constant  relop===  const=1  OutDataTypeStr=boolean
  Compare To Constant5 : simulink/Logic and Bit Operations/Compare To Constant  relop===  const=2  OutDataTypeStr=boolean
  Data Store Read17 : DataStoreRead  DataStoreName=POS_M5
  Data Store Read19 : DataStoreRead  DataStoreName=POS_S15
  Data Store Read20 : DataStoreRead  DataStoreName=POS_S25
  Data Store Write4 : DataStoreWrite  DataStoreName=POS_M5
  Data Store Write6 : DataStoreWrite  DataStoreName=POS_S15
  Data Store Write7 : DataStoreWrite  DataStoreName=POS_S25
  Data Type Conversion1 : DataTypeConversion
  OR : Logic  Operator=OR  AllPortsSameDT=off  OutDataTypeStr=boolean
  OR1 : Logic  Operator=OR  AllPortsSameDT=off  OutDataTypeStr=boolean
  Switch1 : Switch  Criteria=u2 > Threshold
  Switch2 : Switch  Criteria=u2 > Threshold
  Switch3 : Switch  Criteria=u2 > Threshold
  Output : Outport
  Disp1 : Outport  Port=2
  Disp2 : Outport  Port=3
  Disp3 : Outport  Port=4
  wires:
  Compare To Constant5/1 -> AND2/2
  Compare To Constant2/1 -> AND2/1
  AND2/1 -> OR1/1
  AND1/1 -> OR/1
  Compare To Constant4/1 -> AND1/2
  Compare To Constant1/1 -> AND1/1
  TT1/1 -> Compare To Constant3/1, Compare To Constant4/1, Compare To Constant5/1
  Compare To Constant3/1 -> AND/2
  Compare To Constant/1 -> AND/1
  AND/1 -> Switch1/2
  MS22/1 -> OR1/2
  MS11/1 -> OR/2
  OR1/1 -> Switch3/2
  OR/1 -> Switch2/2
  In2/1 -> Switch3/1, Switch2/1, Switch1/1
  In1/1 -> Data Type Conversion1/1, Output/1
  Data Store Read17/1 -> Switch1/3
  Data Store Read19/1 -> Switch2/3
  Switch1/1 -> Data Store Write4/1, Disp1/1
  Switch3/1 -> Data Store Write7/1, Disp3/1
  Data Store Read20/1 -> Switch3/3
  Switch2/1 -> Data Store Write6/1, Disp2/1
  Data Type Conversion1/1 -> Compare To Constant1/1, Compare To Constant2/1, Compare To Constant/1
